simulink model "SignalProcessing"  (R2016b)
settings: Solver=FixedStepDiscrete  StartTime=0.0  StopTime=0.3  RelTol=1e-3
libraries: dspsigops x6, simulink x5, dspsrcs4 x1
settings Model: Creator=Ege  LastModifiedBy=Ege
settings SolverCC: AutoInsertRateTranBlk=on
settings DataIOCC: LimitDataPoints=on  SaveOutput=off  SignalLogging=off  SaveTime=off
settings OptimizationCC: LifeSpan=inf
settings DebuggingCC: AlgebraicLoopMsg=error  SingleTaskRateTransMsg=error  AllowSymbolicDim=off  SFUnexpectedBacktrackingDiag=warning  SFNoUnconditionalDefaultTransitionDiag=warning  SFExecutionAtInitializationDiag=none
settings GRTTargetCC: TargetLangStandard=C89/C90 (ANSI)  GeneratePreprocessorConditionals=Disable all

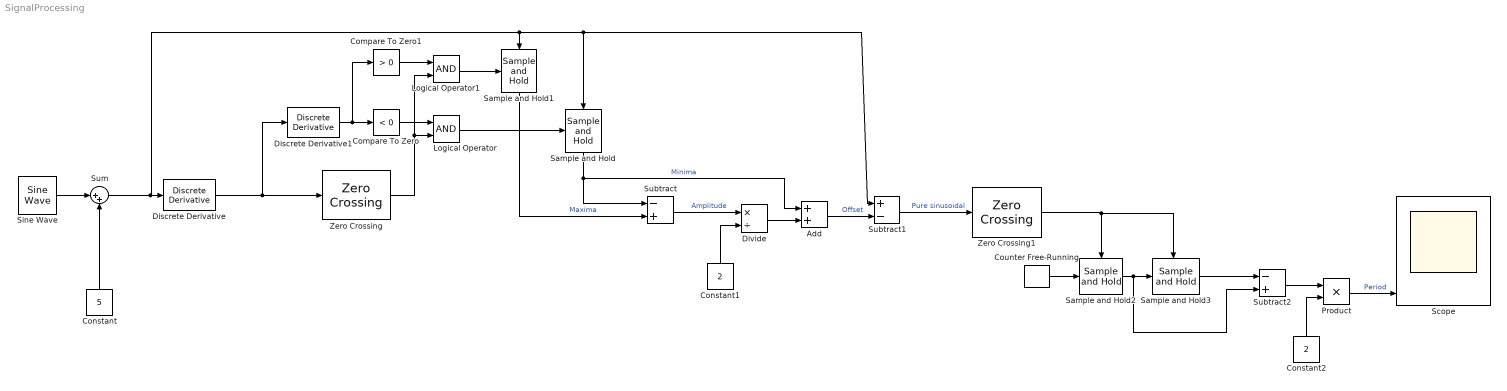
== system SignalProcessing ==
  Add : Sum
  Compare To Zero : simulink/Logic and Bit Operations/Compare To Zero  relop=<  OutDataTypeStr=boolean
  Compare To Zero1 : simulink/Logic and Bit Operations/Compare To Zero  relop=>  OutDataTypeStr=boolean
  Constant : Constant  Value=5
  Constant1 : Constant  Value=2
  Constant2 : Constant  Value=2
  Counter Free-Running : simulink/Sources/Counter Free-Running  NumBits=16  tsamp=-1
  Discrete Derivative : simulink/Discrete/Discrete Derivative  gainval=1.0  ICPrevScaledInput=0.0  OutMin=[]  OutMax=[]  OutDataType=fixdt(1, 16)  OutScaling=2^-10  DoSatur=off
  Discrete Derivative1 : simulink/Discrete/Discrete Derivative  gainval=1.0  ICPrevScaledInput=0.0  OutMin=[]  OutMax=[]  OutDataType=fixdt(1, 16)  OutScaling=2^-10  DoSatur=off
  Divide : Product  Inputs=*/  SaturateOnIntegerOverflow=on  RndMeth=Zero
  Logical Operator : Logic  AllPortsSameDT=off  OutDataTypeStr=boolean
  Logical Operator1 : Logic  AllPortsSameDT=off  OutDataTypeStr=boolean
  Product : Product
  Sample and Hold : dspsigops/Sample and Hold  trig=Rising edge  initCond=0  latchinput=off
  Sample and Hold1 : dspsigops/Sample and Hold  trig=Rising edge  initCond=0  latchinput=off
  Sample and Hold2 : dspsigops/Sample and Hold  trig=Rising edge  initCond=0  latchinput=off
  Sample and Hold3 : dspsigops/Sample and Hold  trig=Rising edge  initCond=0  latchinput=on
  Scope : Scope  NumInputPorts=5
  Sine Wave : dspsrcs4/Sine Wave  Amplitude=1  Frequency=100  Phase=0  SampleMode=Discrete  OutComplex=Real  CompMethod=Trigonometric fcn  TableSize=Speed  SampleTime=1/10000  SamplesPerFrame=1  ResetState=Restart at time zero  OutputFrames=off  dataType=double  wordLen=16  udDataType=sfix(16)  fracBitsMode=Best precision  numFracBits=15  OutDataTypeStr=double  LastOutDataTypeStr=double
  Subtract : Sum  Inputs=-+
  Subtract1 : Sum  Inputs=+-
  Subtract2 : Sum  Inputs=-+  AccumDataTypeStr=fixdt(0,16,0)
  Sum : Sum  Inputs=|++
  Zero Crossing : dspsigops/Zero Crossing  InputProcessing=Columns as channels (frame based)
  Zero Crossing1 : dspsigops/Zero Crossing  InputProcessing=Columns as channels (frame based)
  wires:
  Sine Wave/1 -> Sum/1
  Constant/1 -> Sum/2
  Discrete Derivative/1 -> Discrete Derivative1/1, Zero Crossing/1
  Sample and Hold/1 -> Add/1, Subtract/1  "Minima"
  Compare To Zero/1 -> Logical Operator/1
  Logical Operator/1 -> Sample and Hold/Trigger
  Zero Crossing/1 -> Logical Operator/2, Logical Operator1/2
  Discrete Derivative1/1 -> Compare To Zero1/1, Compare To Zero/1
  Compare To Zero1/1 -> Logical Operator1/1
  Logical Operator1/1 -> Sample and Hold1/Trigger
  Sum/1 -> Sample and Hold1/1, Subtract1/1, Sample and Hold/1, Discrete Derivative/1
  Sample and Hold1/1 -> Subtract/2  "Maxima"
  Subtract/1 -> Divide/1  "Amplitude"
  Constant1/1 -> Divide/2
  Divide/1 -> Add/2
  Add/1 -> Subtract1/2  "Offset"
  Subtract1/1 -> Zero Crossing1/1  "Pure sinusoidal"
  Sample and Hold2/1 -> Subtract2/2, Sample and Hold3/1
  Counter Free-Running/1 -> Sample and Hold2/1
  Zero Crossing1/1 -> Sample and Hold3/Trigger, Sample and Hold2/Trigger
  Sample and Hold3/1 -> Subtract2/1
  Subtract2/1 -> Product/1
  Constant2/1 -> Product/2
  Product/1 -> Scope/5  "Period"
  ? -> Scope/4
